simulink model "NewCAN_4"  (R2021a)
settings: Solver=VariableStepAuto  StartTime=0.0  StopTime=5  RelTol=1e-2
values from neighbouring files (symbols this model uses):
  C = 1e-12    [newmain.m]
  Kidd1 = 0    [newmain.m]
  Kidi1 = 20    [newmain.m]
  Kidi2 = 20    [newmain.m]
  Kidp1 = 5    [newmain.m]
  Kiqd1 = 0    [newmain.m]
  Kiqi1 = 20    [newmain.m]
  Kiqi2 = 20    [newmain.m]
  Kiqp1 = 5    [newmain.m]
  Kiqp2 = 5    [newmain.m]
  Kvdd = 0    [newmain.m]
  Kvdi = 40    [newmain.m]
  Kvdp = 10    [newmain.m]
  Kvqd = 0    [newmain.m]
  Kvqi = 40    [newmain.m]
  Kvqp = 10    [newmain.m]
  L = 100e-3    (= 0.1)    [newmain.m]
  Lf = 4e-3    (= 0.004)    [newmain.m]
  Ll = 31e-6    (= 3.1e-05)    [newmain.m]
  R = 4.33    [newmain.m]
  Rf = 40e-3    (= 0.04)    [newmain.m]
  RL = 0.1    [newmain.m]
  Rl = 0.1    [newmain.m]
  Ts = 0.51e-5    (= 5.1e-06)    [newmain.m]
undefined symbols (not defined in the file or in its folder): Ion, Lithium, sigbuilder_block
libraries: spsMeanLib x48, spsSeriesRLCBranchLib x13, pid_lib x12, spsFirstOrderFilterLib x8, spsIGBTDiodeLib x8, spsPWMGeneratorDCDCLib x8, spsabctodq0Lib x6, spsThreePhaseSeriesRLCBranchLib x4, spsThreePhaseVIMeasurementLib x4, truetime x3, spsdq0toAlphaBetaZeroLib x2, spsSVPWMGenerator2LevelLib x2
(part 1 of 3)
settings Model: SimulationMode=accelerator  OrderedModelArguments=off  Creator=Mori  LastModifiedBy=Mori

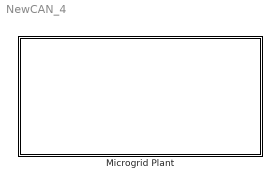
== system NewCAN_4 ==
  Microgrid Plant : Subsystem

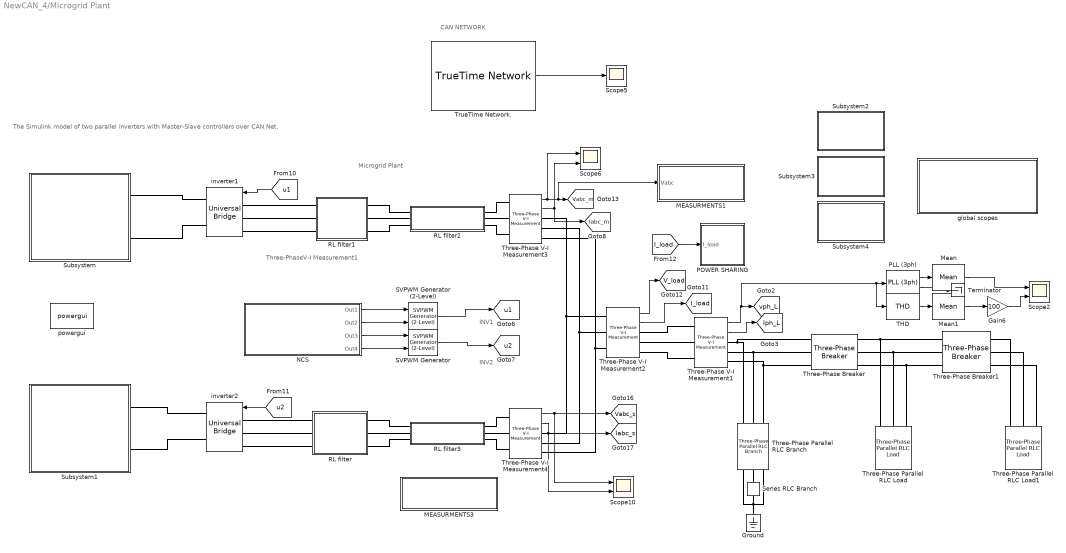
== system NewCAN_4/Microgrid Plant ==
  note: Microgrid Plant
  note: Three-PhaseV-I Measurement1
  note: INV1
  note: INV2
  note: CAN NETWORK
  note: The Simulink model of two parallel inverters with Master-Slave
      | controllers over CAN Net.
  Gain6 : Gain  Gain=100
  Ground : spsGroundLib/Ground  LConnTagsString=a
  MEASURMENTS1 : Subsystem
  MEASURMENTS3 : Subsystem
  Mean : spsMeanLib/Mean  Freq=60  Vinit=0  Ts=0
  Mean1 : spsMeanLib/Mean  Freq=60  Vinit=0  Ts=0
  NCS : Subsystem
  PLL (3ph) : spsPLL3phLib/PLL (3ph)  Fmin=45  Par_Init=[0, 50]  ParK=[180, 3200, 1]  TcD=1e-4  MaxRateChangeFreq=12  FilterCutOffFreq=100  Ts=0  AGC=on
  POWER SHARING : Subsystem
  "RL filter  " : Subsystem
  RL filter1 : Subsystem
  RL filter2 : Subsystem
  RL filter3 : Subsystem
  "SVPWM Generator " : spsSVPWMGenerator2LevelLib/SVPWM Generator (2-Level)  InputType=alpha-beta components  SwitchingPattern=Pattern #1  Fc=6000  ParUref=[0.8 0 50]  Ts=0
      settings: SourceProductBaseCode=PS
  SVPWM Generator (2-Level) : spsSVPWMGenerator2LevelLib/SVPWM Generator (2-Level)  InputType=alpha-beta components  SwitchingPattern=Pattern #1  Fc=6000  ParUref=[0.8 0 50]  Ts=0
      settings: SourceProductBaseCode=PS
  Scope10 : Scope  NumInputPorts=2
  Scope2 : Scope  NumInputPorts=2
  Scope5 : Scope
  Scope6 : Scope  NumInputPorts=2
  Series RLC Branch : spsSeriesRLCBranchLib/Series RLC Branch  LConnTagsString=__new0  RConnTagsString=__new0  BranchType=R  Resistance=Rl  Inductance=1e-3  SetiL0=off  InitialCurrent=0  Capacitance=1e-6  Setx0=off  InitialVoltage=0  Measurements=None
  Subsystem : Subsystem
  Subsystem1 : Subsystem
  Subsystem2 : Subsystem
  Subsystem3 : Subsystem
  Subsystem4 : Subsystem
  THD : spsTHDLib/THD  Freq=50  Ts=0
      settings: SourceProductBaseCode=PS
  Terminator : Terminator
  Three-Phase Parallel RLC Branch : spsThreePhaseParallelRLCBranchLib/Three-Phase Parallel RLC Branch  LConnTagsString=A|B|C  RConnTagsString=A|B|C  BranchType=RLC  Resistance=R  Inductance=L  Capacitance=C  Measurements=None
      settings: SourceProductBaseCode=PS
  Three-Phase Parallel RLC Load : spsThreePhaseParallelRLCLoadLib/Three-Phase Parallel RLC Load  LConnTagsString=A|B|C  Configuration=Y (grounded)  NominalVoltage=380  Vabc=[1e3 1e3 1e3]  Vabcp=[1e3 1e3 1e3]  NominalFrequency=50  UnbalancedPower=off  ActivePower=30e3  InductivePower=5e3  CapacitivePower=0  Pabc=[10e3 9e3 11e3]  QLabc=[100 90 110]  QCabc=[100 90 110]  Pabcp=[10e3 9e3 11e3]  QLabcp=[100 90 110]  QCabcp=[100 90 110]  Measurements=None  LoadType=constant PQ
  Three-Phase Parallel RLC Load1 : spsThreePhaseParallelRLCLoadLib/Three-Phase Parallel RLC Load  LConnTagsString=A|B|C  Configuration=Y (grounded)  NominalVoltage=380  Vabc=[1e3 1e3 1e3]  Vabcp=[1e3 1e3 1e3]  NominalFrequency=50  UnbalancedPower=off  ActivePower=10e3  InductivePower=0  CapacitivePower=0  Pabc=[10e3 9e3 11e3]  QLabc=[100 90 110]  QCabc=[100 90 110]  Pabcp=[10e3 9e3 11e3]  QLabcp=[100 90 110]  QCabcp=[100 90 110]  Measurements=None  LoadType=constant PQ
  Three-Phase V-I Measurement1 : spsThreePhaseVIMeasurementLib/Three-Phase V-I Measurement  VoltageMeasurement=phase-to-ground  SetLabelV=off  LabelV=Vabc  Vpu=off  VpuLL=off  CurrentMeasurement=yes  SetLabelI=off  LabelI=Iabc  Ipu=off  Pbase=100e6  Vbase=500e3  OutputType=Complex  PhasorSimulation=off  PSBequivalent=0
  Three-Phase V-I Measurement2 : spsThreePhaseVIMeasurementLib/Three-Phase V-I Measurement  VoltageMeasurement=phase-to-phase  SetLabelV=off  LabelV=Vabc  Vpu=off  VpuLL=off  CurrentMeasurement=yes  SetLabelI=off  LabelI=Iabc  Ipu=off  Pbase=100e6  Vbase=500e3  OutputType=Complex  PhasorSimulation=off  PSBequivalent=0
  Three-Phase V-I Measurement3 : spsThreePhaseVIMeasurementLib/Three-Phase V-I Measurement  VoltageMeasurement=phase-to-ground  SetLabelV=off  LabelV=Vabc  Vpu=off  VpuLL=off  CurrentMeasurement=yes  SetLabelI=off  LabelI=Iabc  Ipu=off  Pbase=100e6  Vbase=500e3  OutputType=Complex  PhasorSimulation=off  PSBequivalent=0
  Three-Phase V-I Measurement4 : spsThreePhaseVIMeasurementLib/Three-Phase V-I Measurement  VoltageMeasurement=phase-to-ground  SetLabelV=off  LabelV=Vabc  Vpu=off  VpuLL=off  CurrentMeasurement=yes  SetLabelI=off  LabelI=Iabc  Ipu=off  Pbase=100e6  Vbase=500e3  OutputType=Complex  PhasorSimulation=off  PSBequivalent=0
  Three-Phase Breaker : spsThreePhaseBreakerLib/Three-Phase Breaker  InitialState=open  SwitchA=on  SwitchB=on  SwitchC=on  SwitchTimes=[1,4]  External=off  BreakerResistance=0.001  SnubberResistance=1e6  SnubberCapacitance=inf  Measurements=None
  Three-Phase Breaker1 : spsThreePhaseBreakerLib/Three-Phase Breaker  InitialState=open  SwitchA=on  SwitchB=on  SwitchC=on  SwitchTimes=[2,3]  External=off  BreakerResistance=0.001  SnubberResistance=1e6  SnubberCapacitance=inf  Measurements=None
  TrueTime Network. : truetime/TrueTime Network  nwtype=CSMA/AMP (CAN)  nwnbr=1  nnodes=1  rate=10000000  minsize=512  lossprob=0  seed=0  bandwidths=[0.5 0.5]  slotsize=512  schedule=[1 1 2]  memsize=80000  buftype=Common buffer  overflow=Retransmit  dynSchedule=0  miniSlotSize=0  NIT=0  QSortMode=FIFO  sync=0  irtSchedule=0  nrtLength=0  nodeGraph=0  scheduleoutput=on
  global scopes : Subsystem
  inverter1 : spsUniversalBridgeLib/Universal Bridge  Arms=3  SnubberResistance=1e3  SnubberCapacitance=inf  Device=MOSFET / Diodes  Ron=1e-3  Lon=0  ForwardVoltages="[  0  0  ]"  ForwardVoltage=0  GTOparameters=[ 10e-6 , 20e-6 ]  IGBTparameters=[ 1e-6 , 2e-6 ]  Measurements=None  Measurements_2=None  converterType=Rectifier
  inverter2 : spsUniversalBridgeLib/Universal Bridge  Arms=3  SnubberResistance=1e3  SnubberCapacitance=inf  Device=MOSFET / Diodes  Ron=1e-3  Lon=0  ForwardVoltages="[  0  0  ]"  ForwardVoltage=0  GTOparameters=[ 10e-6 , 20e-6 ]  IGBTparameters=[ 1e-6 , 2e-6 ]  Measurements=None  Measurements_2=None  converterType=Rectifier
  powergui : spspowerguiLib/powergui  Priority=1  SimulationMode=Discrete  SampleTime=Ts  frequency=50  Iterations=50  frequencyindice=0  Pbase=100e6  ErrMax=1e-4  UnitsV=kV  UnitsW=MW  buscounter=0  FunctionMessages=off  echomessages=off  EnableUseOfTLC=off  CurrentSourceSwitches=off  DisableSnubberDevices=off  DisableRonSwitches=off  DisableVfSwitches=off  DisplayEquations=off  AutomaticDiscreteSolvers=off  SolverType=Tustin/Backward Euler (TBE)  Interpol=off  ExternalGateDelay=off  methode=on  Ts=10  x0status=blocks  SPID=off  SwTol=0  HookPort=off  NonlinearTolerance=1e-4  nMaxIteration=100  ContinueOnMaxIteration=off  RestoreLinks=warning  ResistiveCurrentMeasurement=off  Frange=[0:2:50]  Ylog=off  Xlog=off  ShowGrid=on  save=off  variable=ZData  structure=Inverter2  ZoomFFT=off  StartTime=0.075  cycles=1  DisplayStyle=2  fundamental=50  FreqAxis=off  MaxFrequency=50*400  frequencyindicesteady=1  RmsSteady=1  display=off
  tag scope: I_load=global, Iabc_m=global, Iabc_s=global, Iph_L=global, V_load=global, Vabc_m=global, Vabc_s=global, u1=global, u2=global, vph_L=global
  wires:
  [u1] -> inverter1/1
  [u2] -> inverter2/1
  Three-Phase V-I Measurement3/2 -> [Iabc_m], Scope6/2
  Three-Phase V-I Measurement4/1 -> Scope10/1, [Vabc_s]
  Three-Phase V-I Measurement4/2 -> Scope10/2, [Iabc_s]
  Three-Phase V-I Measurement2/1 -> [V_load]
  Three-Phase V-I Measurement2/2 -> [I_load]
  NCS/2(Out2) -> SVPWM Generator (2-Level)/2
  SVPWM Generator (2-Level)/1 -> [u1]
  NCS/3(Out3) -> "SVPWM Generator "/1
  NCS/4(Out4) -> "SVPWM Generator "/2
  "SVPWM Generator "/1 -> [u2]
  NCS/1(Out1) -> SVPWM Generator (2-Level)/1
  TrueTime Network./1 -> Scope5/1
  Three-Phase V-I Measurement3/1 -> Scope6/1, MEASURMENTS1/1(Vabc), [Vabc_m]
  [I_load] -> POWER SHARING/1(I_load)
  Three-Phase V-I Measurement1/2 -> [Iph_L]
  PLL (3ph)/1 -> Mean/1
  Three-Phase V-I Measurement1/1 -> [vph_L], THD/1, PLL (3ph)/1
  PLL (3ph)/2 -> Terminator/1
  Mean/1 -> Scope2/1
  THD/1 -> Mean1/1
  Gain6/1 -> Scope2/2
  Mean1/1 -> Gain6/1
  connections:
  "RL filter  "/LConn2 -- inverter2/LConn2
  RL filter1/LConn2 -- inverter1/LConn2
  Three-Phase V-I Measurement2/LConn3 -- Three-Phase V-I Measurement4/RConn3 -- Three-Phase V-I Measurement3/RConn3
  RL filter1/LConn1 -- inverter1/LConn1
  RL filter1/LConn3 -- inverter1/LConn3
  "RL filter  "/LConn1 -- inverter2/LConn1
  Three-Phase V-I Measurement2/LConn2 -- Three-Phase V-I Measurement4/RConn2 -- Three-Phase V-I Measurement3/RConn2
  "RL filter  "/LConn3 -- inverter2/LConn3
  Three-Phase V-I Measurement1/LConn1 -- Three-Phase V-I Measurement2/RConn1
  Three-Phase V-I Measurement1/LConn2 -- Three-Phase V-I Measurement2/RConn2
  Three-Phase V-I Measurement1/LConn3 -- Three-Phase V-I Measurement2/RConn3
  Three-Phase V-I Measurement2/LConn1 -- Three-Phase V-I Measurement4/RConn1 -- Three-Phase V-I Measurement3/RConn1
  Subsystem/RConn1 -- inverter1/RConn1
  inverter1/RConn2 -- Subsystem/RConn2
  Series RLC Branch/LConn1 -- Three-Phase Parallel RLC Branch/RConn2
  Ground/LConn1 -- Series RLC Branch/RConn1 -- Three-Phase Parallel RLC Branch/RConn3 -- Three-Phase Parallel RLC Branch/RConn1
  RL filter2/LConn2 -- RL filter1/RConn2
  RL filter2/LConn1 -- RL filter1/RConn1
  RL filter2/LConn3 -- RL filter1/RConn3
  Three-Phase V-I Measurement3/LConn3 -- RL filter2/RConn3
  Three-Phase V-I Measurement3/LConn2 -- RL filter2/RConn2
  Three-Phase V-I Measurement3/LConn1 -- RL filter2/RConn1
  Three-Phase V-I Measurement4/LConn1 -- RL filter3/RConn1
  Three-Phase V-I Measurement4/LConn2 -- RL filter3/RConn2
  Three-Phase V-I Measurement4/LConn3 -- RL filter3/RConn3
  RL filter3/LConn2 -- "RL filter  "/RConn2
  RL filter3/LConn1 -- "RL filter  "/RConn1
  RL filter3/LConn3 -- "RL filter  "/RConn3
  Subsystem1/RConn2 -- inverter2/RConn2
  inverter2/RConn1 -- Subsystem1/RConn1
  Three-Phase V-I Measurement1/RConn1 -- Three-Phase Breaker/LConn1 -- Three-Phase Parallel RLC Branch/LConn1
  Three-Phase V-I Measurement1/RConn2 -- Three-Phase Breaker/LConn2 -- Three-Phase Parallel RLC Branch/LConn2
  Three-Phase V-I Measurement1/RConn3 -- Three-Phase Breaker/LConn3 -- Three-Phase Parallel RLC Branch/LConn3
  Three-Phase Breaker1/LConn2 -- Three-Phase Parallel RLC Load/LConn2 -- Three-Phase Breaker/RConn2
  Three-Phase Breaker1/LConn3 -- Three-Phase Parallel RLC Load/LConn3 -- Three-Phase Breaker/RConn3
  Three-Phase Parallel RLC Load/LConn1 -- Three-Phase Breaker/RConn1 -- Three-Phase Breaker1/LConn1
  Three-Phase Parallel RLC Load1/LConn3 -- Three-Phase Breaker1/RConn3
  Three-Phase Parallel RLC Load1/LConn1 -- Three-Phase Breaker1/RConn1
  Three-Phase Parallel RLC Load1/LConn2 -- Three-Phase Breaker1/RConn2

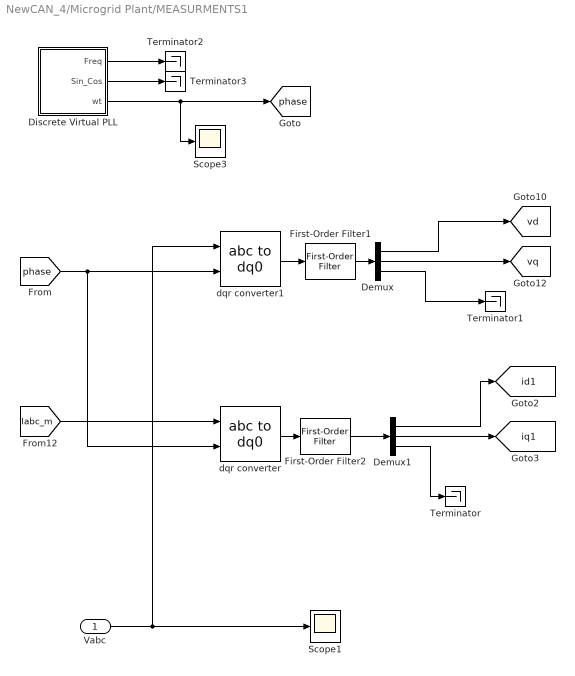
== system NewCAN_4/Microgrid Plant/MEASURMENTS1 ==
  Vabc : Inport
  Demux : Demux  Outputs=3
  Demux1 : Demux  Outputs=3
  Discrete Virtual PLL : Subsystem  DialogController=POWERSYS.PowerSysDialog  mask(Discrete Virtual PLL){Freq=50, Phase=0, Ts=Ts}
      mask prompts: Freq "Frequency (Hz):"; Phase "Phase (degrees):"; Ts "Sample time:"
      mask help:
      | This virtual PLL has no input signal. The block simulates the outputs of an actual PLL by  using the parameters specified in the mask.
      |
      | Output 1: Frequency (Hz)
      | Output 2: Vectorized output  [sin(wt)  cos(wt)]
      | Output 3: wt in rad/s (varying from 0 to 2*pi)
      mask init:
      | power_initmask();
      mask Display: disp('')
  First-Order Filter1 : spsFirstOrderFilterLib/First-Order Filter  FilterType=Lowpass  Tc=1e-3  Ts=0  Initialize=off  Vac_Init=[0, 0, 60]  Vdc_Init=0  PlotResponse=off  FreqRange="[0,  200,  1]"
  First-Order Filter2 : spsFirstOrderFilterLib/First-Order Filter  FilterType=Lowpass  Tc=1e-3  Ts=0  Initialize=off  Vac_Init=[0, 0, 60]  Vdc_Init=0  PlotResponse=off  FreqRange="[0,  200,  1]"
  Scope1 : Scope
  Scope3 : Scope
  Terminator{,1..3} (4 alike) : Terminator
  dqr converter : spsabctodq0Lib/abc to dq0  Alignment=Aligned with phase A axis
  dqr converter1 : spsabctodq0Lib/abc to dq0  Alignment=Aligned with phase A axis
  tag scope: id1=global, iq1=global, phase=global, vd=global, vq=global
  wires:
  Vabc/1 -> dqr converter1/1, Scope1/1
  [phase] -> dqr converter/2, dqr converter1/2
  dqr converter1/1 -> First-Order Filter1/1
  dqr converter/1 -> First-Order Filter2/1
  Demux/3 -> Terminator1/1
  Demux/2 -> [vq]
  Demux/1 -> [vd]
  Demux1/1 -> [id1]
  Demux1/2 -> [iq1]
  Demux1/3 -> Terminator/1
  Discrete Virtual PLL/3(wt) -> [phase], Scope3/1
  Discrete Virtual PLL/2(Sin_Cos) -> Terminator3/1
  Discrete Virtual PLL/1(Freq) -> Terminator2/1
  [Iabc_m] -> dqr converter/1
  First-Order Filter1/1 -> Demux/1
  First-Order Filter2/1 -> Demux1/1

== system NewCAN_4/Microgrid Plant/MEASURMENTS3 ==
  Demux : Demux  Outputs=3
  Demux1 : Demux  Outputs=3
  First-Order Filter1 : spsFirstOrderFilterLib/First-Order Filter  FilterType=Lowpass  Tc=1e-3  Ts=0  Initialize=off  Vac_Init=[0, 0, 60]  Vdc_Init=0  PlotResponse=off  FreqRange="[0,  200,  1]"
  First-Order Filter2 : spsFirstOrderFilterLib/First-Order Filter  FilterType=Lowpass  Tc=1e-3  Ts=0  Initialize=off  Vac_Init=[0, 0, 60]  Vdc_Init=0  PlotResponse=off  FreqRange="[0,  200,  1]"
  Scope3 : Scope
  Scope5 : Scope
  Terminator : Terminator
  Terminator1 : Terminator
  abc to dq1 : spsabctodq0Lib/abc to dq0  Alignment=Aligned with phase A axis
  abc to dq3 : spsabctodq0Lib/abc to dq0  Alignment=Aligned with phase A axis
  tag scope: id2=global, iq2=global, vd_s=global, vq_s=global
  wires:
  Demux/2 -> [iq2]
  [phase] -> abc to dq3/2, abc to dq1/2
  Demux/1 -> [id2]
  abc to dq3/1 -> Scope5/1, First-Order Filter1/1
  [Iabc_s] -> abc to dq3/1, Scope3/1
  Demux/3 -> Terminator/1
  [Vabc_s] -> abc to dq1/1
  Demux1/3 -> Terminator1/1
  abc to dq1/1 -> First-Order Filter2/1
  Demux1/1 -> [vd_s]
  Demux1/2 -> [vq_s]
  First-Order Filter1/1 -> Demux/1
  First-Order Filter2/1 -> Demux1/1

== system NewCAN_4/Microgrid Plant/NCS ==
  Master controller : Subsystem
  Transformations : Subsystem
  slave controller : Subsystem
  Out1 : Outport
  Out2 : Outport  Port=2
  Out3 : Outport  Port=3
  Out4 : Outport  Port=4
  wires:
  Transformations/1(Out2) -> Out1/1
  Transformations/4(Out4) -> Out4/1
  Transformations/3(Out5) -> Out3/1
  Transformations/2(Out1) -> Out2/1
  [dd2] -> Transformations/3(dd2)
  [dq1] -> Transformations/2(dq1)
  [dd1] -> Transformations/1(dd1)
  [dq2] -> Transformations/4(dq2)

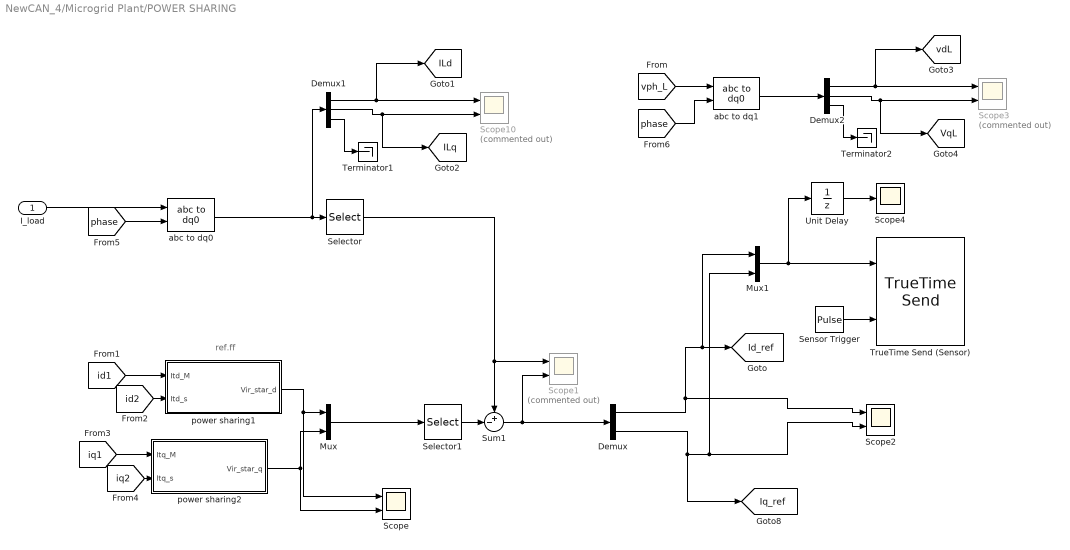
== system NewCAN_4/Microgrid Plant/POWER SHARING ==
  note: ref.ff
  I_load : Inport
  Demux : Demux  Outputs=2
  Demux1 : Demux  Outputs=3
  Demux2 : Demux  Outputs=3
  Mux : Mux  Inputs=2
  Mux1 : Mux  Inputs=2
  Scope : Scope  NumInputPorts=2
  Scope1 : Scope  Commented=on  NumInputPorts=2
  Scope10 : Scope  Commented=on  NumInputPorts=2
  Scope2 : Scope  NumInputPorts=2
  Scope3 : Scope  Commented=on  NumInputPorts=2
  Scope4 : Scope
  Selector : Selector  InputPortWidth=3  IndexOptions=Index vector (dialog)  Indices=[1 2]  OutputSizes=1
  Selector1 : Selector  InputPortWidth=2  IndexOptions=Index vector (dialog)  Indices=[1 2]  OutputSizes=1
  Sensor Trigger : DiscretePulseGenerator  PulseType=Time based  Period=1/10000  PulseWidth=25
  Sum1 : Sum  Inputs=+-|
  Terminator1 : Terminator
  Terminator2 : Terminator
  TrueTime Send (Sensor) : truetime/TrueTime Send  trigger=rising  nwnbr=1  sender=1  indim=2  recsource=internal  receiver=1  lengthsource=internal  length=512  priosource=internal  prio=1  msgIDsource=internal  msgID=0  dynamicSegment=dynamic
  Unit Delay : UnitDelay  InputProcessing=Columns as channels (frame based)  SampleTime=0.21e-3  HasFrameUpgradeWarning=on
  abc to dq0 : spsabctodq0Lib/abc to dq0  Alignment=Aligned with phase A axis
  abc to dq1 : spsabctodq0Lib/abc to dq0  Alignment=Aligned with phase A axis
  power sharing1 : MATLAB Function  TreatAsAtomicUnit=on
  power sharing2 : MATLAB Function  TreatAsAtomicUnit=on
  tag scope: ILd=global, ILq=global, Id_ref=global, Iq_ref=global, VqL=global, vdL=global
  wires:
  I_load/1 -> abc to dq0/1
  [phase] -> abc to dq0/2
  power sharing1/1(Vir_star_d) -> Mux/1, Scope/1
  power sharing2/1(Vir_star_q) -> Scope/2, Mux/2
  Sum1/1 -> Scope1/2, Demux/1
  Selector1/1 -> Sum1/2
  Demux1/1 -> [ILd], Scope10/1
  Demux1/2 -> [ILq], Scope10/2
  Demux1/3 -> Terminator1/1
  Demux/2 -> [Iq_ref], Scope2/2, Mux1/2
  Demux/1 -> Scope2/1, Mux1/1, [Id_ref]
  [id1] -> power sharing1/1(Itd_M)
  [id2] -> power sharing1/2(Itd_s)
  [iq1] -> power sharing2/1(Itq_M)
  [iq2] -> power sharing2/2(Itq_s)
  Selector/1 -> Scope1/1, Sum1/1
  Mux/1 -> Selector1/1
  Sensor Trigger/1 -> TrueTime Send (Sensor)/2
  abc to dq0/1 -> Demux1/1, Selector/1
  [vph_L] -> abc to dq1/1
  [phase] -> abc to dq1/2
  Demux2/3 -> Terminator2/1
  abc to dq1/1 -> Demux2/1
  Demux2/2 -> Scope3/2, [VqL]
  Demux2/1 -> Scope3/1, [vdL]
  Mux1/1 -> Unit Delay/1, TrueTime Send (Sensor)/1
  Unit Delay/1 -> Scope4/1

== system NewCAN_4/Microgrid Plant/RL filter   ==
  Three-Phase Series RLC Branch : spsThreePhaseSeriesRLCBranchLib/Three-Phase Series RLC Branch  LConnTagsString=A|B|C  RConnTagsString=A|B|C  BranchType=RL  Resistance=Rf  Inductance=Lf  Capacitance=C  Measurements=None
  Connection Port : PMIOPort  Side=Left
  Connection Port1 : PMIOPort  Port=2  Side=Left
  Connection Port2 : PMIOPort  Port=3  Side=Left
  Connection Port4 : PMIOPort  Port=4  Side=Right
  Connection Port3 : PMIOPort  Port=5  Side=Right
  Connection Port5 : PMIOPort  Port=6  Side=Right
  connections:
  Three-Phase Series RLC Branch/RConn2 -- Connection Port4/RConn1
  Connection Port3/RConn1 -- Three-Phase Series RLC Branch/RConn1
  Connection Port5/RConn1 -- Three-Phase Series RLC Branch/RConn3
  Connection Port1/RConn1 -- Three-Phase Series RLC Branch/LConn2
  Connection Port2/RConn1 -- Three-Phase Series RLC Branch/LConn3
  Connection Port/RConn1 -- Three-Phase Series RLC Branch/LConn1

== system NewCAN_4/Microgrid Plant/RL filter1 ==
  Three-Phase Series RLC Branch : spsThreePhaseSeriesRLCBranchLib/Three-Phase Series RLC Branch  LConnTagsString=A|B|C  RConnTagsString=A|B|C  BranchType=RL  Resistance=Rf  Inductance=Lf  Capacitance=C  Measurements=None
  Connection Port : PMIOPort  Side=Left
  Connection Port1 : PMIOPort  Port=2  Side=Left
  Connection Port2 : PMIOPort  Port=3  Side=Left
  Connection Port4 : PMIOPort  Port=4  Side=Right
  Connection Port3 : PMIOPort  Port=5  Side=Right
  Connection Port5 : PMIOPort  Port=6  Side=Right
  connections:
  Connection Port/RConn1 -- Three-Phase Series RLC Branch/LConn1
  Connection Port1/RConn1 -- Three-Phase Series RLC Branch/LConn2
  Three-Phase Series RLC Branch/LConn3 -- Connection Port2/RConn1
  Three-Phase Series RLC Branch/RConn3 -- Connection Port5/RConn1
  Connection Port4/RConn1 -- Three-Phase Series RLC Branch/RConn2
  Connection Port3/RConn1 -- Three-Phase Series RLC Branch/RConn1

== system NewCAN_4/Microgrid Plant/RL filter2 ==
  Three-Phase Series RLC Branch : spsThreePhaseSeriesRLCBranchLib/Three-Phase Series RLC Branch  LConnTagsString=A|B|C  RConnTagsString=A|B|C  BranchType=RL  Resistance=RL  Inductance=Ll  Capacitance=C  Measurements=None
  Connection Port : PMIOPort  Side=Left
  Connection Port1 : PMIOPort  Port=2  Side=Left
  Connection Port2 : PMIOPort  Port=3  Side=Left
  Connection Port4 : PMIOPort  Port=4  Side=Right
  Connection Port3 : PMIOPort  Port=5  Side=Right
  Connection Port5 : PMIOPort  Port=6  Side=Right
  connections:
  Three-Phase Series RLC Branch/RConn1 -- Connection Port3/RConn1
  Three-Phase Series RLC Branch/RConn2 -- Connection Port4/RConn1
  Connection Port5/RConn1 -- Three-Phase Series RLC Branch/RConn3
  Three-Phase Series RLC Branch/LConn3 -- Connection Port2/RConn1
  Connection Port1/RConn1 -- Three-Phase Series RLC Branch/LConn2
  Connection Port/RConn1 -- Three-Phase Series RLC Branch/LConn1

== system NewCAN_4/Microgrid Plant/RL filter3 ==
  Three-Phase Series RLC Branch : spsThreePhaseSeriesRLCBranchLib/Three-Phase Series RLC Branch  LConnTagsString=A|B|C  RConnTagsString=A|B|C  BranchType=RL  Resistance=RL  Inductance=Ll  Capacitance=C  Measurements=None
  Connection Port : PMIOPort  Side=Left
  Connection Port1 : PMIOPort  Port=2  Side=Left
  Connection Port2 : PMIOPort  Port=3  Side=Left
  Connection Port4 : PMIOPort  Port=4  Side=Right
  Connection Port3 : PMIOPort  Port=5  Side=Right
  Connection Port5 : PMIOPort  Port=6  Side=Right
  connections:
  Connection Port/RConn1 -- Three-Phase Series RLC Branch/LConn1
  Connection Port1/RConn1 -- Three-Phase Series RLC Branch/LConn2
  Three-Phase Series RLC Branch/LConn3 -- Connection Port2/RConn1
  Three-Phase Series RLC Branch/RConn3 -- Connection Port5/RConn1
  Connection Port4/RConn1 -- Three-Phase Series RLC Branch/RConn2
  Connection Port3/RConn1 -- Three-Phase Series RLC Branch/RConn1

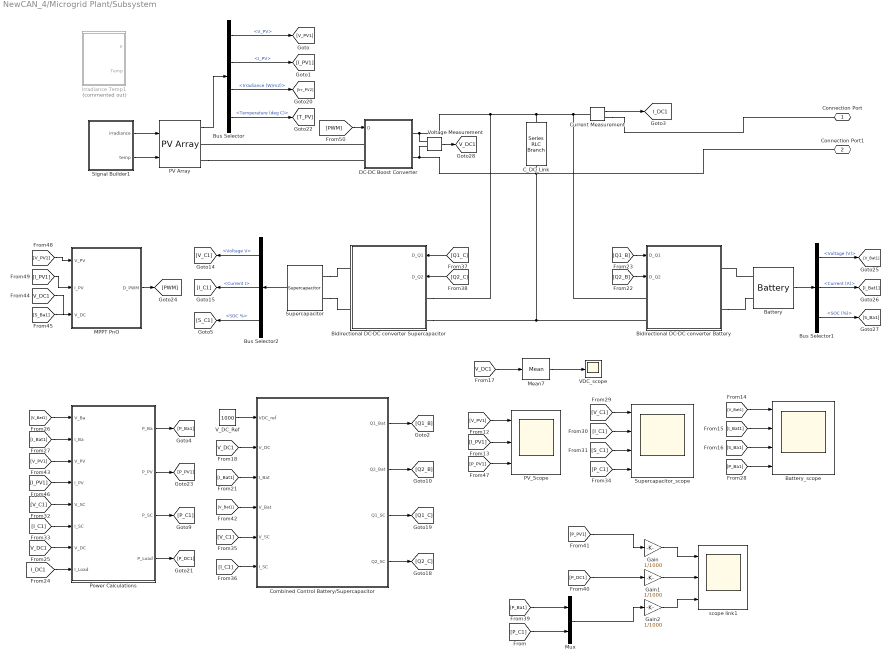
== system NewCAN_4/Microgrid Plant/Subsystem ==
  Battery : spsBatteryLib/Battery  BatType=Lithium-Ion  ShowTempParam=off  ThermalPreset=no  ShowAgeParam=off  NomV=583  NomQ=14  SOC=50  Batt_Tr=0.2  PresetModel=on  MaxQ=14  MinV=437.25  FullV=678.6045  Dis_rate=6.087  R=0.41643  Normal_OP=12.6609  expZone="[629.865     0.6878261]"  current=[6.5 13 32.5]  Units=Time  Tci=20  NomT=20  T2=-30  MaxQ2=4.8  FullV2=7.1  Normal_OP2=5.655  expZone2="[6.58           1]"  Rca=0.6  ti=2000  Dp=0  Neq0=0  Tsim=1e6  Ta1=25  Qeol=5.4*0.9  Reol=0.013333*1.2  Char_age=[2.3478, 3]  Dis_age=[2.3478, 10]  N1=1500  N2=10500  N3=1000  N4=1400  Ta2=45  N5=950
  "Battery_scope " : Scope  NumInputPorts=4
  Bidirectional DC-DC converter Battery : Subsystem
  Bidirectional DC-DC converter Supercapacitor : Subsystem
  Bus Selector : BusSelector  OutputSignals=V_PV,I_PV,Irradiance (W/m2),Temperature (deg C)
  Bus Selector1 : BusSelector  OutputSignals=Voltage (V),Current (A),SOC (%)
  Bus Selector2 : BusSelector  OutputSignals=Voltage V,Current I,SOC %
  C_DC_Link : spsSeriesRLCBranchLib/Series RLC Branch  LConnTagsString=__new0  RConnTagsString=__new0  BranchType=C  Resistance=1  Inductance=1e-3  SetiL0=off  InitialCurrent=0  Capacitance=300e-6  Setx0=off  InitialVoltage=0  Measurements=None
  Combined Control Battery/Supercapacitor : Subsystem
  Current Measurement : spsCurrentMeasurementLib/Current Measurement  PhasorSimulation=off  OutputType=Complex  PSBequivalent=0
  DC-DC Boost Converter : Subsystem
  Gain : Gain  Gain=1/1000
  Gain1 : Gain  Gain=1/1000
  Gain2 : Gain  Gain=1/1000
  Irradiance Temp1 : Subsystem  Tag=STV Subsys  Commented=on  LoadFcn=sigbuilder_block('load');  StartFcn=sigbuilder_block('start');  StopFcn=sigbuilder_block('stop');  ClipboardFcn=sigbuilder_block('clipboard');  mask(Sigbuilder block){tuvar=[0:10]}
      mask help: Sigbuilder GUI
      mask init:
      | if ~strcmp(get_param(bdroot(gcbh),'SimulationStatus'),'stopped') tuvar = sigbuilder_block('maskInit'); end
      settings: CopyFcn=sigbuilder_block('copy');  DeleteFcn=sigbuilder_block('delete');  ModelCloseFcn=sigbuilder_block('modelClose');  PreSaveFcn=sigbuilder_block('preSave');  PauseFcn=sigbuilder_block('pause')  ContinueFcn=sigbuilder_block('continue')  NameChangeFcn=sigbuilder_block('namechange');  OpenFcn=sigbuilder_block('open',[216.75 117 531.75 395.25 ]);  CloseFcn=sigbuilder_block('close');
      mask Display: plot(0, 0, 100, 100,[2, 2, 32, 32, 2], [68, 8, 8, 68, 68],[32, 2], [38, 38], [32, 19, 2],[53, 60, 44], [32, 17, 17, 2],[16, 16, 31, 31]);txt = getActiveGroup(gcbh);text(2, 100, txt,'verticalAlignment', 'top');
  MPPT PnO : Subsystem
  Mean7 : spsMeanLib/Mean  Freq=60  Vinit=0  Ts=0
  Mux : Mux  Inputs=2
  PV Array : spsPVArrayLib/PV Array  Npar=6  Nser=30  PlotType=array @ 25 deg.C & specified irradiances  S_vec="[ 1000 800 500  250 ]"  Temp_C_vec="[0 25 50  ]"  ModuleName=Yingli Energy (China) YL250P-29b  PlotWhenSelected=on  Pm=250.496  Ncell=60  Voc=38.4  Isc=8.79  Vm=30.4  Im=8.24  beta_Voc_pc=-0.337  alpha_Isc_pc=0.0438  beta_Voc=-0.12941  alpha_Isc=0.00385  IL=8.8005  I0=1.272e-10  nI=0.99849  Rsh=362.5163  Rs=0.42475  RobustModel=off  RobustCellTemperature=313.3991  BAL=on  Tc=Tc  Tfilter=5e-5
  PV_Scope : Scope  NumInputPorts=3
  Power Calculations : Subsystem
  Signal Builder1 : Subsystem  Tag=STV Subsys  LoadFcn=sigbuilder_block('load');  StartFcn=sigbuilder_block('start');  StopFcn=sigbuilder_block('stop');  ClipboardFcn=sigbuilder_block('clipboard');  mask(Sigbuilder block){tuvar=[0:10]}
      mask help: Simulink:masks:SigbuilderBlock_MD
      mask init:
      | if ~strcmp(get_param(bdroot(gcbh),'SimulationStatus'),'stopped') tuvar = sigbuilder_block('maskInit'); end
      settings: CopyFcn=sigbuilder_block('copy');  DeleteFcn=sigbuilder_block('delete');  ModelCloseFcn=sigbuilder_block('modelClose');  PreSaveFcn=sigbuilder_block('preSave');  PauseFcn=sigbuilder_block('pause');  ContinueFcn=sigbuilder_block('continue');  NameChangeFcn=sigbuilder_block('namechange');  OpenFcn=sigbuilder_block('open',[6 0 1012.5 477.75 ]);  CloseFcn=sigbuilder_block('close');
      mask Display: plot(0, 0, 100, 100,[2, 2, 32, 32, 2], [68, 8, 8, 68, 68],[32, 2], [38, 38], [32, 19, 2],[53, 60, 44], [32, 17, 17, 2],[16, 16, 31, 31]);txt = getActiveGroup(gcbh);text(2, 100, txt,'verticalAlignment', 'top');
  Supercapacitor : spsSupercapacitorLib/Supercapacitor  C=210  Rdc=0.003  Voltage=850  Ns=1  Np=1  Vinit=850  Temp=25  PresetModel=off  EstParam=off  Nc=1  r=1e-9  epsilon=6.0208e-10  Ich=10  Vstern="[0.161  2.7  7.8]"  Self_dis=on  Ioc=10  Vself="[980  975  970  965]"  demandeplot=off  I="[10  20 100  500]"  Units=sec  Vmax=0  If=0  deltaV=0  alpha=0  sec=0
      settings: SourceProductBaseCode=PS
  Supercapacitor_scope : Scope  NumInputPorts=4
  VDC_scope : Scope
  V_DC_Ref : Constant  Value=1000
  Voltage Measurement : spsVoltageMeasurementLib/Voltage Measurement  PhasorSimulation=off  OutputType=Complex  PSBequivalent=0
  scope link1 : Scope  NumInputPorts=3
  Connection Port : PMIOPort  Side=Right
  Connection Port1 : PMIOPort  Port=2  Side=Right
  tag scope: I_DC1=global, V_DC1=global
  wires:
  [V_C1] -> Power Calculations/5(V_SC)
  [V_C1] -> Combined Control Battery/Supercapacitor/5("V_SC ")
  [I_C1] -> Combined Control Battery/Supercapacitor/6(I_SC)
  Bus Selector2/1 -> [V_C1]  "<Voltage V>"
  [V_PV1] -> PV_Scope/1
  Mux/1 -> Gain2/1
  [S_C1] -> Supercapacitor_scope/3
  [V_Bat1] -> "Battery_scope "/1
  [P_Ba1] -> Mux/1
  [V_Bat1] -> Combined Control Battery/Supercapacitor/4(V_Bat)
  Mean7/1 -> VDC_scope/1
  [V_DC1] -> Combined Control Battery/Supercapacitor/2(V_DC)
  Voltage Measurement/1 -> [V_DC1]
  [S_Ba1] -> "Battery_scope "/3
  Bus Selector1/3 -> [S_Ba1]  "<SOC (%)>"
  Bus Selector1/2 -> [I_Bat1]  "<Current (A)>"
  [I_Bat1] -> Power Calculations/2(I_Ba)
  [I_Bat1] -> "Battery_scope "/2
  [V_Bat1] -> Power Calculations/1(V_Ba)
  Bus Selector/4 -> [T_PV]  "<Temperature (deg C)>"
  [PWM] -> DC-DC Boost Converter/1(D)
  [P_DC1] -> Gain1/1
  [V_DC1] -> Mean7/1
  [Q2_C] -> Bidirectional DC-DC converter Supercapacitor/2(D_Q2)
  [I_Bat1] -> Combined Control Battery/Supercapacitor/3(I_Bat)
  [P_PV1] -> Gain/1
  [I_C1] -> Supercapacitor_scope/2
  [I_C1] -> Power Calculations/6(I_SC)
  [P_Ba1] -> "Battery_scope "/4
  [V_DC1] -> Power Calculations/7(V_DC)
  Battery/1 -> Bus Selector1/1
  Power Calculations/4(P_Load) -> [P_DC1]
  [Q2_B] -> Bidirectional DC-DC converter Battery/2(D_Q2)
  PV Array/1 -> Bus Selector/1
  [S_Ba1] -> ?
  Combined Control Battery/Supercapacitor/4(Q2_SC) -> [Q2_C]
  [Q1_C] -> Bidirectional DC-DC converter Supercapacitor/1(D_Q1)
  [P_PV1] -> PV_Scope/3
  [Q1_B] -> Bidirectional DC-DC converter Battery/1(D_Q1)
  Combined Control Battery/Supercapacitor/2(Q2_Bat) -> [Q2_B]
  Supercapacitor/1 -> Bus Selector2/1
  Bus Selector2/3 -> [S_C1]  "<SOC %>"
  [I_PV1] -> PV_Scope/2
  Current Measurement/1 -> [I_DC1]
  [P_C1] -> Supercapacitor_scope/4
  Power Calculations/1(P_Ba) -> [P_Ba1]
  [I_DC1] -> Power Calculations/8(I_Load)
  [V_PV1] -> MPPT PnO/1(V_PV)
  V_DC_Ref/1 -> Combined Control Battery/Supercapacitor/1(VDC_ref)
  [V_PV1] -> Power Calculations/3(V_PV)
  [V_DC1] -> MPPT PnO/3(V_DC)
  Bus Selector1/1 -> [V_Bat1]  "<Voltage (V)>"
  Power Calculations/2(P_PV) -> [P_PV1]
  Combined Control Battery/Supercapacitor/1(Q1_Bat) -> [Q1_B]
  [I_PV1] -> Power Calculations/4(I_PV)
  Bus Selector/2 -> [I_PV1]  "<I_PV>"
  [I_PV1] -> MPPT PnO/2(I_PV)
  MPPT PnO/1(D_PWM) -> [PWM]
  Power Calculations/3(P_SC) -> [P_C1]
  Combined Control Battery/Supercapacitor/3(Q1_SC) -> [Q1_C]
  [P_C1] -> Mux/2
  Bus Selector/1 -> [V_PV1]  "<V_PV>"
  Bus Selector/3 -> [Irr_PV2]  "<Irradiance (W/m2)>"
  [V_C1] -> Supercapacitor_scope/1
  Bus Selector2/2 -> [I_C1]  "<Current I>"
  Signal Builder1/1(irradiance) -> PV Array/1
  Signal Builder1/2(temp) -> PV Array/2
  Gain/1 -> scope link1/1
  Gain1/1 -> scope link1/2
  Gain2/1 -> scope link1/3
  connections:
  Current Measurement/LConn1 -- DC-DC Boost Converter/RConn1 -- Voltage Measurement/LConn1 -- Bidirectional DC-DC converter Supercapacitor/LConn1 -- C_DC_Link/LConn1 -- Bidirectional DC-DC converter Battery/LConn1
  DC-DC Boost Converter/LConn1 -- PV Array/RConn1
  Bidirectional DC-DC converter Battery/LConn2 -- Connection Port1/RConn1 -- C_DC_Link/RConn1 -- Voltage Measurement/LConn2 -- DC-DC Boost Converter/RConn2 -- Bidirectional DC-DC converter Supercapacitor/LConn2
  Supercapacitor/LConn2 -- Bidirectional DC-DC converter Supercapacitor/RConn2
  PV Array/RConn2 -- DC-DC Boost Converter/LConn2
  Bidirectional DC-DC converter Battery/RConn2 -- Battery/LConn2
  Current Measurement/RConn1 -- Connection Port/RConn1
  Supercapacitor/LConn1 -- Bidirectional DC-DC converter Supercapacitor/RConn1
  Battery/LConn1 -- Bidirectional DC-DC converter Battery/RConn1

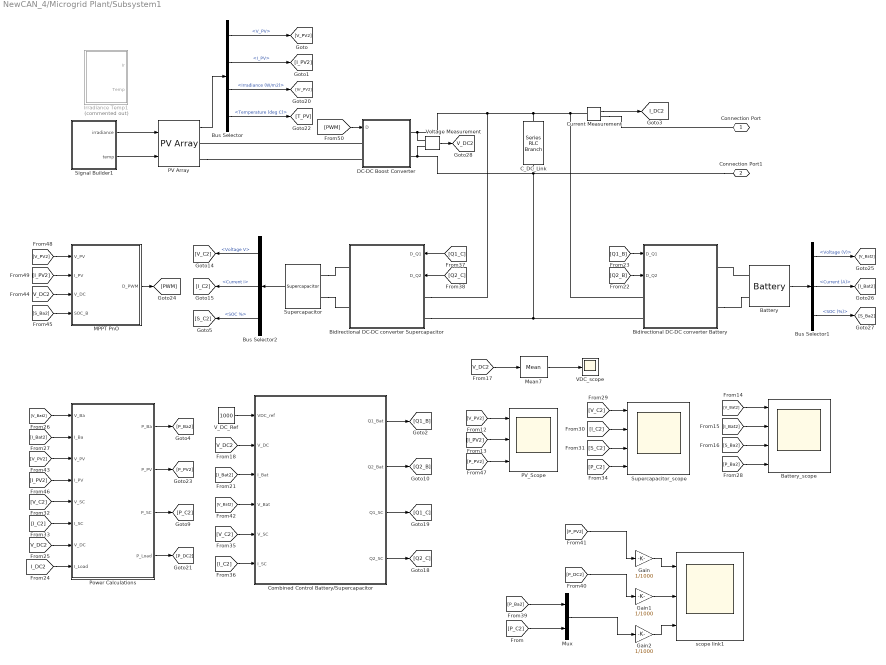
== system NewCAN_4/Microgrid Plant/Subsystem1 ==
  Battery : spsBatteryLib/Battery  BatType=Lithium-Ion  ShowTempParam=off  ThermalPreset=no  ShowAgeParam=off  NomV=583  NomQ=10  SOC=50  Batt_Tr=0.2  PresetModel=on  MaxQ=10  MinV=437.25  FullV=678.6045  Dis_rate=4.3478  R=0.583  Normal_OP=9.0435  expZone="[629.865     0.4913043]"  current=[4.5 7 11.5]  Units=Time  Tci=20  NomT=20  T2=-30  MaxQ2=4.8  FullV2=7.1  Normal_OP2=5.655  expZone2="[6.58           1]"  Rca=0.6  ti=2000  Dp=0  Neq0=0  Tsim=1e6  Ta1=25  Qeol=5.4*0.9  Reol=0.013333*1.2  Char_age=[2.3478, 3]  Dis_age=[2.3478, 10]  N1=1500  N2=10500  N3=1000  N4=1400  Ta2=45  N5=950
  "Battery_scope " : Scope  NumInputPorts=4
  Bidirectional DC-DC converter Battery : Subsystem
  Bidirectional DC-DC converter Supercapacitor : Subsystem
  Bus Selector : BusSelector  OutputSignals=V_PV,I_PV,Irradiance (W/m2),Temperature (deg C)
  Bus Selector1 : BusSelector  OutputSignals=Voltage (V),Current (A),SOC (%)
  Bus Selector2 : BusSelector  OutputSignals=Voltage V,Current I,SOC %
  C_DC_Link : spsSeriesRLCBranchLib/Series RLC Branch  LConnTagsString=__new0  RConnTagsString=__new0  BranchType=C  Resistance=1  Inductance=1e-3  SetiL0=off  InitialCurrent=0  Capacitance=300e-6  Setx0=off  InitialVoltage=0  Measurements=None
  Combined Control Battery/Supercapacitor : Subsystem
  Current Measurement : spsCurrentMeasurementLib/Current Measurement  PhasorSimulation=off  OutputType=Complex  PSBequivalent=0
  DC-DC Boost Converter : Subsystem
  Gain : Gain  Gain=1/1000
  Gain1 : Gain  Gain=1/1000
  Gain2 : Gain  Gain=1/1000
  Irradiance Temp1 : Subsystem  Tag=STV Subsys  Commented=on  LoadFcn=sigbuilder_block('load');  StartFcn=sigbuilder_block('start');  StopFcn=sigbuilder_block('stop');  ClipboardFcn=sigbuilder_block('clipboard');  mask(Sigbuilder block){tuvar=[0:10]}
      mask help: Sigbuilder GUI
      mask init:
      | if ~strcmp(get_param(bdroot(gcbh),'SimulationStatus'),'stopped') tuvar = sigbuilder_block('maskInit'); end
      settings: CopyFcn=sigbuilder_block('copy');  DeleteFcn=sigbuilder_block('delete');  ModelCloseFcn=sigbuilder_block('modelClose');  PreSaveFcn=sigbuilder_block('preSave');  PauseFcn=sigbuilder_block('pause')  ContinueFcn=sigbuilder_block('continue')  NameChangeFcn=sigbuilder_block('namechange');  OpenFcn=sigbuilder_block('open',[216.75 117 531.75 395.25 ]);  CloseFcn=sigbuilder_block('close');
      mask Display: plot(0, 0, 100, 100,[2, 2, 32, 32, 2], [68, 8, 8, 68, 68],[32, 2], [38, 38], [32, 19, 2],[53, 60, 44], [32, 17, 17, 2],[16, 16, 31, 31]);txt = getActiveGroup(gcbh);text(2, 100, txt,'verticalAlignment', 'top');
  MPPT PnO : Subsystem
  Mean7 : spsMeanLib/Mean  Freq=60  Vinit=0  Ts=0
  Mux : Mux  Inputs=2
  PV Array : spsPVArrayLib/PV Array  Npar=3  Nser=30  PlotType=array @ 25 deg.C & specified irradiances  S_vec="[ 1000 800 500  250 ]"  Temp_C_vec="[0 25 50  ]"  ModuleName=Yingli Energy (China) YL250C-30b  PlotWhenSelected=on  Pm=252.815  Ncell=60  Voc=37.6  Isc=9.1  Vm=29.5  Im=8.57  beta_Voc_pc=-0.3  alpha_Isc_pc=0.044  beta_Voc=-0.1128  alpha_Isc=0.004004  IL=9.111  I0=3.084e-11  nI=0.92381  Rsh=475.5958  Rs=0.45532  RobustModel=off  RobustCellTemperature=313.3991  BAL=on  Tc=Tc  Tfilter=5e-5
  PV_Scope : Scope  NumInputPorts=3
  Power Calculations : Subsystem
  Signal Builder1 : Subsystem  Tag=STV Subsys  LoadFcn=sigbuilder_block('load');  StartFcn=sigbuilder_block('start');  StopFcn=sigbuilder_block('stop');  ClipboardFcn=sigbuilder_block('clipboard');  mask(Sigbuilder block){tuvar=[0:10]}
      mask help: Simulink:masks:SigbuilderBlock_MD
      mask init:
      | if ~strcmp(get_param(bdroot(gcbh),'SimulationStatus'),'stopped') tuvar = sigbuilder_block('maskInit'); end
      settings: CopyFcn=sigbuilder_block('copy');  DeleteFcn=sigbuilder_block('delete');  ModelCloseFcn=sigbuilder_block('modelClose');  PreSaveFcn=sigbuilder_block('preSave');  PauseFcn=sigbuilder_block('pause');  ContinueFcn=sigbuilder_block('continue');  NameChangeFcn=sigbuilder_block('namechange');  OpenFcn=sigbuilder_block('open',[6 0 1012.5 477.75 ]);  CloseFcn=sigbuilder_block('close');
      mask Display: plot(0, 0, 100, 100,[2, 2, 32, 32, 2], [68, 8, 8, 68, 68],[32, 2], [38, 38], [32, 19, 2],[53, 60, 44], [32, 17, 17, 2],[16, 16, 31, 31]);txt = getActiveGroup(gcbh);text(2, 100, txt,'verticalAlignment', 'top');
  Supercapacitor : spsSupercapacitorLib/Supercapacitor  C=50  Rdc=0.0028  Voltage=820  Ns=1  Np=1  Vinit=820  Temp=25  PresetModel=off  EstParam=off  Nc=1  r=1e-9  epsilon=6.0208e-10  Ich=10  Vstern="[0.161  2.7  7.8]"  Self_dis=on  Ioc=10  Vself="[980  975  970  965]"  demandeplot=off  I="[10  20 100  500]"  Units=sec  Vmax=0  If=0  deltaV=0  alpha=0  sec=0
      settings: SourceProductBaseCode=PS
  Supercapacitor_scope : Scope  NumInputPorts=4
  VDC_scope : Scope
  V_DC_Ref : Constant  Value=1000
  Voltage Measurement : spsVoltageMeasurementLib/Voltage Measurement  PhasorSimulation=off  OutputType=Complex  PSBequivalent=0
  scope link1 : Scope  NumInputPorts=3
  Connection Port : PMIOPort  Side=Right
  Connection Port1 : PMIOPort  Port=2  Side=Right
  tag scope: I_DC2=global, V_DC2=global
  wires:
  Bus Selector2/2 -> [I_C2]  "<Current I>"
  [V_C2] -> Supercapacitor_scope/1
  Bus Selector/3 -> [Irr_PV2]  "<Irradiance (W/m2)>"
  Bus Selector/1 -> [V_PV2]  "<V_PV>"
  [P_C2] -> Mux/2
  Combined Control Battery/Supercapacitor/3(Q1_SC) -> [Q1_C]
  Power Calculations/3(P_SC) -> [P_C2]
  MPPT PnO/1(D_PWM) -> [PWM]
  [I_PV2] -> MPPT PnO/2(I_PV)
  Bus Selector/2 -> [I_PV2]  "<I_PV>"
  [I_PV2] -> Power Calculations/4(I_PV)
  Combined Control Battery/Supercapacitor/1(Q1_Bat) -> [Q1_B]
  Power Calculations/2(P_PV) -> [P_PV2]
  Bus Selector1/1 -> [V_Bat2]  "<Voltage (V)>"
  [V_DC2] -> MPPT PnO/3(V_DC)
  [V_PV2] -> Power Calculations/3(V_PV)
  V_DC_Ref/1 -> Combined Control Battery/Supercapacitor/1(VDC_ref)
  [V_PV2] -> MPPT PnO/1(V_PV)
  [I_DC2] -> Power Calculations/8(I_Load)
  Power Calculations/1(P_Ba) -> [P_Ba2]
  [P_C2] -> Supercapacitor_scope/4
  Current Measurement/1 -> [I_DC2]
  [I_PV2] -> PV_Scope/2
  Bus Selector2/3 -> [S_C2]  "<SOC %>"
  Supercapacitor/1 -> Bus Selector2/1
  Combined Control Battery/Supercapacitor/2(Q2_Bat) -> [Q2_B]
  [Q1_B] -> Bidirectional DC-DC converter Battery/1(D_Q1)
  [P_PV2] -> PV_Scope/3
  [Q1_C] -> Bidirectional DC-DC converter Supercapacitor/1(D_Q1)
  Combined Control Battery/Supercapacitor/4(Q2_SC) -> [Q2_C]
  [S_Ba2] -> MPPT PnO/4(SOC_B)
  PV Array/1 -> Bus Selector/1
  [Q2_B] -> Bidirectional DC-DC converter Battery/2(D_Q2)
  Power Calculations/4(P_Load) -> [P_DC2]
  Battery/1 -> Bus Selector1/1
  [V_DC2] -> Power Calculations/7(V_DC)
  [P_Ba2] -> "Battery_scope "/4
  [I_C2] -> Power Calculations/6(I_SC)
  [I_C2] -> Supercapacitor_scope/2
  [P_PV2] -> Gain/1
  [I_Bat2] -> Combined Control Battery/Supercapacitor/3(I_Bat)
  [Q2_C] -> Bidirectional DC-DC converter Supercapacitor/2(D_Q2)
  [V_DC2] -> Mean7/1
  [P_DC2] -> Gain1/1
  [PWM] -> DC-DC Boost Converter/1(D)
  Bus Selector/4 -> [T_PV]  "<Temperature (deg C)>"
  [V_Bat2] -> Power Calculations/1(V_Ba)
  [I_Bat2] -> "Battery_scope "/2
  [I_Bat2] -> Power Calculations/2(I_Ba)
  Bus Selector1/2 -> [I_Bat2]  "<Current (A)>"
  Bus Selector1/3 -> [S_Ba2]  "<SOC (%)>"
  [S_Ba2] -> "Battery_scope "/3
  Voltage Measurement/1 -> [V_DC2]
  [V_DC2] -> Combined Control Battery/Supercapacitor/2(V_DC)
  Mean7/1 -> VDC_scope/1
  [V_Bat2] -> Combined Control Battery/Supercapacitor/4(V_Bat)
  [P_Ba2] -> Mux/1
  [V_Bat2] -> "Battery_scope "/1
  [S_C2] -> Supercapacitor_scope/3
  Mux/1 -> Gain2/1
  [V_PV2] -> PV_Scope/1
  Bus Selector2/1 -> [V_C2]  "<Voltage V>"
  [I_C2] -> Combined Control Battery/Supercapacitor/6(I_SC)
  [V_C2] -> Combined Control Battery/Supercapacitor/5("V_SC ")
  [V_C2] -> Power Calculations/5(V_SC)
  Signal Builder1/1(irradiance) -> PV Array/1
  Signal Builder1/2(temp) -> PV Array/2
  Gain/1 -> scope link1/1
  Gain1/1 -> scope link1/2
  Gain2/1 -> scope link1/3
  connections:
  Battery/LConn1 -- Bidirectional DC-DC converter Battery/RConn1
  Supercapacitor/LConn1 -- Bidirectional DC-DC converter Supercapacitor/RConn1
  Current Measurement/RConn1 -- Connection Port/RConn1
  Bidirectional DC-DC converter Battery/RConn2 -- Battery/LConn2
  PV Array/RConn2 -- DC-DC Boost Converter/LConn2
  Supercapacitor/LConn2 -- Bidirectional DC-DC converter Supercapacitor/RConn2
  Connection Port1/RConn1 -- Bidirectional DC-DC converter Battery/LConn2 -- Bidirectional DC-DC converter Supercapacitor/LConn2 -- DC-DC Boost Converter/RConn2 -- Voltage Measurement/LConn2 -- C_DC_Link/RConn1
  DC-DC Boost Converter/LConn1 -- PV Array/RConn1
  Current Measurement/LConn1 -- Bidirectional DC-DC converter Battery/LConn1 -- C_DC_Link/LConn1 -- Bidirectional DC-DC converter Supercapacitor/LConn1 -- Voltage Measurement/LConn1 -- DC-DC Boost Converter/RConn1

== system NewCAN_4/Microgrid Plant/Subsystem2 ==
  MATLAB Function : MATLAB Function  TreatAsAtomicUnit=on
  MATLAB Function1 : MATLAB Function  TreatAsAtomicUnit=on
  tag scope: P_L=global, Q_L=global
  wires:
  [vd] -> MATLAB Function/2(Vd), MATLAB Function1/2(Vd)
  MATLAB Function1/1(QL) -> [Q_L]
  MATLAB Function/1(pL) -> [P_L]
  [ILq] -> MATLAB Function1/1(ILq)
  [ILd] -> MATLAB Function/1(ILd)

== system NewCAN_4/Microgrid Plant/Subsystem3 ==
  MATLAB Function : MATLAB Function  TreatAsAtomicUnit=on
  MATLAB Function1 : MATLAB Function  TreatAsAtomicUnit=on
  tag scope: P_M=global, Q_M=global
  wires:
  MATLAB Function/1(p_M) -> [P_M]
  MATLAB Function1/1(Q_M) -> [Q_M]
  [iq1] -> MATLAB Function1/1(Itq_M)
  [vd] -> MATLAB Function1/2(Vd), MATLAB Function/2(Vd)
  [id1] -> MATLAB Function/1(Itd_M)

== system NewCAN_4/Microgrid Plant/Subsystem4 ==
  MATLAB Function : MATLAB Function  TreatAsAtomicUnit=on
  MATLAB Function1 : MATLAB Function  TreatAsAtomicUnit=on
  tag scope: P_S=global, Q_S=global
  wires:
  [id2] -> MATLAB Function/1(Itd_s)
  [vd_s] -> MATLAB Function/2(Vds), MATLAB Function1/2(Vds)
  [iq2] -> MATLAB Function1/1(Itq_s)
  MATLAB Function1/1(Q_S) -> [Q_S]
  MATLAB Function/1(p_S) -> [P_S]

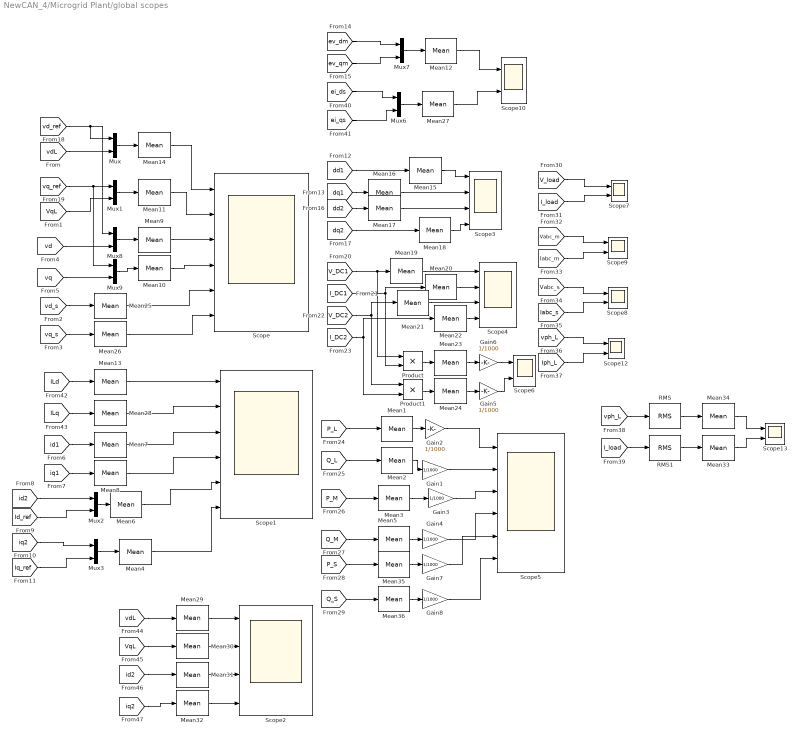
== system NewCAN_4/Microgrid Plant/global scopes ==
  Gain{1..8} (8 alike) : Gain  Gain=1/1000
  Mean{1..28,35..36} (30 alike) : spsMeanLib/Mean  Freq=50  Vinit=0  Ts=0
  Mean{29..34} (6 alike) : spsMeanLib/Mean  Freq=60  Vinit=0  Ts=0
  Mux{,1..3,6..9} (8 alike) : Mux  Inputs=2
  Product : Product
  Product1 : Product
  RMS : spsRMSLib/RMS  TrueRMS=on  Freq=50  RMSInit=0  Ts=0
  RMS1 : spsRMSLib/RMS  TrueRMS=on  Freq=50  RMSInit=0  Ts=0
  Scope : Scope  NumInputPorts=6
  Scope1 : Scope  NumInputPorts=6
  Scope{6..10,12..13} (7 alike) : Scope  NumInputPorts=2
  Scope2 : Scope  NumInputPorts=4
  Scope3 : Scope  NumInputPorts=4
  Scope4 : Scope  NumInputPorts=4
  Scope5 : Scope  NumInputPorts=6
  wires:
  Mux/1 -> Mean14/1
  [vq_ref] -> Mux9/1, Mux1/1
  [VqL] -> Mux1/2
  Mux1/1 -> Mean11/1
  [id1] -> Mean7/1
  [iq1] -> Mean8/1
  [id2] -> Mux2/1
  [Id_ref] -> Mux2/2
  [iq2] -> Mux3/1
  [Iq_ref] -> Mux3/2
  [dd1] -> Mean15/1
  [dq1] -> Mean16/1
  [dd2] -> Mean17/1
  [dq2] -> Mean18/1
  [V_DC1] -> Product/1, Mean19/1
  [I_DC1] -> Product/2, Mean20/1
  [V_DC2] -> Product1/1, Mean21/1
  [I_DC2] -> Mean22/1, Product1/2
  [Q_L] -> Mean2/1
  [P_L] -> Mean1/1
  [P_M] -> Mean3/1
  [Q_M] -> Mean5/1
  [vq_s] -> Mean26/1
  [vd_s] -> Mean25/1
  Mux2/1 -> Mean6/1
  Mux3/1 -> Mean4/1
  [vd_ref] -> Mux8/1, Mux/1
  [vdL] -> Mux/2
  Product/1 -> Mean23/1
  Product1/1 -> Mean24/1
  [Vabc_m] -> Scope9/1
  [Iabc_m] -> Scope9/2
  [Vabc_s] -> Scope8/1
  [Iabc_s] -> Scope8/2
  [V_load] -> Scope7/1
  [I_load] -> Scope7/2
  [vph_L] -> Scope12/1
  [Iph_L] -> Scope12/2
  Mean1/1 -> Gain2/1
  Mean2/1 -> Gain1/1
  Mean5/1 -> Gain4/1
  Mean3/1 -> Gain3/1
  Mean4/1 -> Scope1/6
  Mean6/1 -> Scope1/5
  Mean11/1 -> Scope/2
  Mean14/1 -> Scope/1
  Mean15/1 -> Scope3/1
  Mean16/1 -> Scope3/2
  Mean17/1 -> Scope3/3
  Mean18/1 -> Scope3/4
  Mean19/1 -> Scope4/1
  Mean20/1 -> Scope4/2
  Mean21/1 -> Scope4/3
  Mean22/1 -> Scope4/4
  Mean23/1 -> Gain6/1
  Mean24/1 -> Gain5/1
  [I_load] -> RMS1/1
  [vph_L] -> RMS/1
  Mux6/1 -> Mean27/1
  [ei_qs] -> Mux6/2
  [ei_ds] -> Mux6/1
  [ev_dm] -> Mux7/1
  [ev_qm] -> Mux7/2
  Mux7/1 -> Mean12/1
  Mean27/1 -> Scope10/2
  Mean12/1 -> Scope10/1
  [ILd] -> Mean13/1
  [ILq] -> Mean28/1
  Mean9/1 -> Scope/3
  Mean10/1 -> Scope/4
  Mean7/1 -> Scope1/3
  Mean8/1 -> Scope1/4
  Mean25/1 -> Scope/5
  Mean26/1 -> Scope/6
  Mean13/1 -> Scope1/1
  Mean28/1 -> Scope1/2
  Mux8/1 -> Mean9/1
  [vd] -> Mux8/2
  Mux9/1 -> Mean10/1
  [vq] -> Mux9/2
  Mean30/1 -> Scope2/2
  Mean31/1 -> Scope2/3
  Mean29/1 -> Scope2/1
  [VqL] -> Mean30/1
  Mean32/1 -> Scope2/4
  [vdL] -> Mean29/1
  [iq2] -> Mean32/1
  [id2] -> Mean31/1
  Gain2/1 -> Scope5/1
  Gain1/1 -> Scope5/2
  Gain3/1 -> Scope5/3
  Gain4/1 -> Scope5/4
  Gain6/1 -> Scope6/1
  Gain5/1 -> Scope6/2
  RMS1/1 -> Mean33/1
  RMS/1 -> Mean34/1
  Mean35/1 -> Gain7/1
  Mean36/1 -> Gain8/1
  Gain7/1 -> Scope5/5
  Gain8/1 -> Scope5/6
  [Q_S] -> Mean36/1
  [P_S] -> Mean35/1
  Mean33/1 -> Scope13/2
  Mean34/1 -> Scope13/1

== system NewCAN_4/Microgrid Plant/MEASURMENTS1/Discrete Virtual PLL ==
  note: Pierre Giroux, Gilbert Sybille
      | Power System Simulation Laboratory
      | IREQ, Hydro-Quebc
  note: Discrete Virtual PLL
  Constant4 : Constant  Value=2*pi
  Deg->Rad : Gain  Gain=pi/180  SaturateOnIntegerOverflow=on  OutDataTypeStr=Inherit: Same as input  ParamDataTypeStr=Inherit: Same as input
  Freq1 : Constant  Value=Freq
  Freq2 : Constant  Value=2*pi
  Initial Vd_Vq1 : Constant  Value=Phase
  Math Function : Math  Operator=mod  SignedPower=on  SaturateOnIntegerOverflow=on
  Mux : Mux  Inputs=2
  Product : Product  Inputs=***  InputSameDT=on  SaturateOnIntegerOverflow=on  OutDataTypeStr=Inherit: Same as first input
  Sum : Sum  InputSameDT=on  SaturateOnIntegerOverflow=on  OutDataTypeStr=Inherit: Same as first input
  Trigonometric Function : Trigonometry
  Trigonometric Function1 : Trigonometry  Operator=cos
  t : DigitalClock  SampleTime=Ts
  Freq : Outport  VectorParamsAs1DForOutWhenUnconnected=off
  Sin_Cos : Outport  Port=2  VectorParamsAs1DForOutWhenUnconnected=off
  wt : Outport  Port=3  VectorParamsAs1DForOutWhenUnconnected=off
  wires:
  Sum/1 -> Math Function/1
  t/1 -> Product/2
  Freq2/1 -> Product/3
  Freq1/1 -> Product/1, Freq/1
  Deg->Rad/1 -> Sum/2
  Initial Vd_Vq1/1 -> Deg->Rad/1
  Product/1 -> Sum/1
  Constant4/1 -> Math Function/2
  Math Function/1 -> wt/1, Trigonometric Function1/1, Trigonometric Function/1
  Trigonometric Function/1 -> Mux/1
  Trigonometric Function1/1 -> Mux/2
  Mux/1 -> Sin_Cos/1
